simulink model "non_linear_system_2_2014b"  (R2014b)
settings: Solver=ode3  SolverMode=SingleTasking  StartTime=0.0  StopTime=100  FixedStep=0.001  RelTol=1e-3
values from neighbouring files (symbols this model uses):
  A = double(subs(A, [x; u], [x_equ; u_equ]))    [Second_order_perturbation.m]    (also in main.m)
  amp = 0.3    [Second_order_perturbation.m]    (also in main.m)
  B = double(subs(B, [x; u], [x_equ; u_equ]))    [Second_order_perturbation.m]    (also in main.m)
  u_equ = 0.16    [Second_order_perturbation.m]    (also in main.m)
  x_equ = [0.2; 0]    [Second_order_perturbation.m]    (also in main.m)
settings Model: CovMetricSettings=dwe  CovHtmlReporting=off  covSaveCumulativeToWorkspaceVar=off  CovSaveSingleToWorkspaceVar=off  CovExternalEMLEnable=on  CovSFcnEnable=on  Creator=soren  LastModifiedBy=soren
settings DataIOCC: LimitDataPoints=off  SaveFormat=StructureWithTime  ReturnWorkspaceOutputs=on
settings DebuggingCC: SolverPrmCheckMsg=none  FrameProcessingCompatibilityMsg=error  SFUnexpectedBacktrackingDiag=error  SFNoUnconditionalDefaultTransitionDiag=error
settings HardwareCC: ProdBitPerPointer=64  ProdLargestAtomicFloat=Float  ProdIntDivRoundTo=Zero  ProdEndianess=LittleEndian  ProdHWDeviceType=Specified
settings ModelReferenceCC: PropagateSignalLabelsOutOfModel=on
settings SFSimCC: SimUseLocalCustomCode=on
settings RTWCC: RTWUseLocalCustomCode=on
settings GRTTargetCC: TargetLangStandard=C99 (ISO)

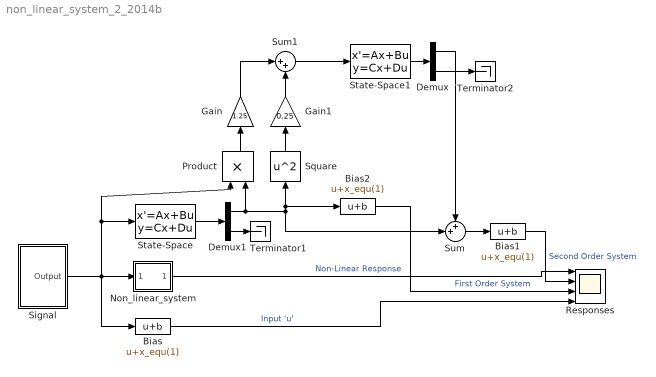
== system non_linear_system_2_2014b ==
  Bias : Bias  Bias=x_equ(1)
  Bias1 : Bias  Bias=x_equ(1)
  Bias2 : Bias  Bias=x_equ(1)
  Demux : Demux  Outputs=2
  Demux1 : Demux  Outputs=2
  Gain : Gain  Gain=1.25
  Gain1 : Gain  Gain=0.25
  Non_linear_system : Subsystem
  Product : Product
  Responses : Scope  NumInputPorts=4
      settings: TimeRange=auto  ShowLegends=on  MaxDataPoints=5000  SaveToWorkspace=off  SaveName=ScopeData  YMin=0.08749~-5~-5~-5  YMax=0.32581~5~5~5  SampleTime=-1
  Signal : Subsystem
  Square : Math  Operator=square  SaturateOnIntegerOverflow=on
  State-Space : StateSpace  A=A  B=B  C=eye(2,2)  D=zeros(2,1)  X0=0
  State-Space1 : StateSpace  A=A  B=B  C=eye(2,2)  D=zeros(2,1)  X0=0
  Sum : Sum  Inputs=++|
  Sum1 : Sum  Inputs=|++
  Terminator1 : Terminator
  Terminator2 : Terminator
  wires:
  Non_linear_system/1(Output) -> Responses/1  "Non-Linear Response"
  Signal/1(Output) -> Non_linear_system/1(Input), Product/1, State-Space/1, Bias/1
  Bias1/1 -> Responses/2  "Second Order System"
  State-Space/1 -> Demux1/1
  Demux1/2 -> Terminator1/1
  Product/1 -> Gain/1
  Square/1 -> Gain1/1
  Gain1/1 -> Sum1/2
  Gain/1 -> Sum1/1
  Sum1/1 -> State-Space1/1
  Sum/1 -> Bias1/1
  State-Space1/1 -> Demux/1
  Demux/1 -> Sum/1
  Demux/2 -> Terminator2/1
  Bias/1 -> Responses/4  "Input 'u'"
  Demux1/1 -> Product/2, Square/1, Bias2/1, Sum/2
  Bias2/1 -> Responses/3  "First Order System"

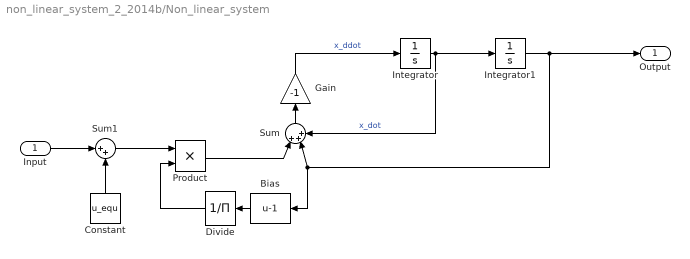
== system non_linear_system_2_2014b/Non_linear_system ==
  Input : Inport
  Bias : Bias  Bias=-1
  Constant : Constant  Value=u_equ
  Divide : Product  Inputs=/
  Gain : Gain  Gain=-1
  Integrator : Integrator
  Integrator1 : Integrator  InitialCondition=x_equ(1)
  Product : Product
  Sum : Sum  Inputs=|+++
  Sum1 : Sum  Inputs=|++
  Output : Outport
  wires:
  Integrator/1 -> Sum/3, Integrator1/1  "x_dot"
  Gain/1 -> Integrator/1  "x_ddot"
  Constant/1 -> Sum1/2
  Input/1 -> Sum1/1
  Integrator1/1 -> Output/1, Bias/1, Sum/2
  Bias/1 -> Divide/1
  Sum/1 -> Gain/1
  Sum1/1 -> Product/1
  Product/1 -> Sum/1
  Divide/1 -> Product/2

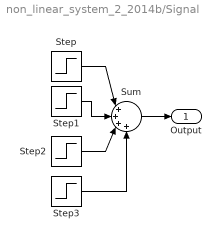
== system non_linear_system_2_2014b/Signal ==
  Step : Step  Time=20  After=0.16*amp  SampleTime=0
  Step1 : Step  Time=40  After=-0.16*amp  SampleTime=0
  Step2 : Step  Time=60  After=-0.16*amp  SampleTime=0
  Step3 : Step  Time=80  After=0.16*amp  SampleTime=0
  Sum : Sum  Inputs=|++++
  Output : Outport
  wires:
  Sum/1 -> Output/1
  Step2/1 -> Sum/3
  Step/1 -> Sum/1
  Step1/1 -> Sum/2
  Step3/1 -> Sum/4
